simulink model "BaseMotorSimX"  (R2020b)
settings: Solver=VariableStepAuto  StartTime=0.0  StopTime=SimTime  FixedStep=solverTimeStep  RelTol=1e-3
InitFcn:
  | StartupScript
StartFcn:
  | StartupScript
values from neighbouring files (symbols this model uses):
  CF = 372.0    (= 372)    [StartupScript.m]
  Isat = 10.0    (= 10)    [StartupScript.m]
  Kb = 800.0    (= 800)    [StartupScript.m]
  Kdb = 1/(Zerob^2) - Kpb/Poleb    (= 0.414500592554)    [StartupScript.m]
  Kib = 1.0    (= 1)    [StartupScript.m]
  Kmb = 23.4*1e-3    (= 0.0234)    [StartupScript.m]
  Kpb = 2/(Zerob) - 1/Poleb    (= 1.28897849462)    [StartupScript.m]
  PidLim = 1024    [StartupScript.m]
  PidUCGain = 5/1024    (= 0.0048828125)    [StartupScript.m]
  r2d = 180/pi    (= 57.2957795131)    [StartupScript.m]
  sensorGain = 150.0    (= 150)    [StartupScript.m]
  SimStepTime = 1e-3    (= 0.001)    [StartupScript.m]
  Vsat = 18.0    (= 18)    [StartupScript.m]
libraries: cstblocks x3
settings Model: Creator=nisch  LastModifiedBy=nisch

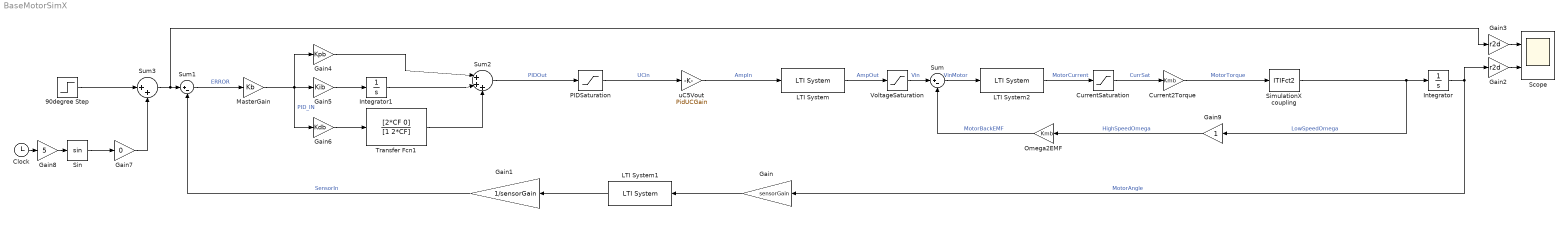
== system BaseMotorSimX ==
  90degree Step : Step  Time=0  After=pi/2  SampleTime=0
  Clock : Clock
  Current2Torque : Gain  Gain=Kmb
  CurrentSaturation : Saturate  UpperLimit=Isat  LowerLimit=-Isat
  Gain : Gain  Gain=sensorGain
  Gain1 : Gain  Gain=1/sensorGain
  Gain2 : Gain  Gain=r2d
  Gain3 : Gain  Gain=r2d
  Gain4 : Gain  Gain=Kpb
  Gain5 : Gain  Gain=Kib
  Gain6 : Gain  Gain=Kdb
  Gain7 : Gain  Gain=0
  Gain8 : Gain  Gain=5
  Gain9 : Gain
  Integrator : Integrator
  Integrator1 : Integrator
  LTI System : cstblocks/LTI System  sys=VoltageAmplifier  IC=[]
  LTI System1 : cstblocks/LTI System  sys=Hs  IC=[]
  LTI System2 : cstblocks/LTI System  sys=Electricalb  IC=[]
  MasterGain : Gain  Gain=Kb
  Omega2EMF : Gain  Gain=Kmb
  PIDSaturation : Saturate  UpperLimit=PidLim  LowerLimit=-PidLim
  Scope : Scope  NumInputPorts=2
  SimulationX coupling : S-Function  FunctionName=ITIFct2  Parameters=ip, port, ts, nIn, nOut  SFunctionDeploymentMode=off  EnableBusSupport=off  mask{ip='localhost', port=4097, ts=SimStepTime, nIn=1, nOut=1}
      mask prompts: ip "Address: ip"; port "Port Number: port [-]"; ts "Communication Step Size: ts [s]"; nIn "Input Vector Dimension (to SimulationX): nIn [-]"; nOut "Output Vector Dimension (from SimulationX): nOut [-]"
      mask help: Coupling Element
  Sin : Trigonometry
  Sum : Sum  Inputs=|+-
  Sum1 : Sum  Inputs=|+-
  Sum2 : Sum  Inputs=|+++
  Sum3 : Sum  Inputs=|++
  Transfer Fcn1 : TransferFcn  Numerator=[2*CF 0]  Denominator=[1 2*CF]
  VoltageSaturation : Saturate  UpperLimit=Vsat  LowerLimit=-Vsat
  uC5Vout : Gain  Gain=PidUCGain
  wires:
  Sum/1 -> LTI System2/1  "VinMotor"
  Omega2EMF/1 -> Sum/2  "MotorBackEMF"
  Sum1/1 -> MasterGain/1  "ERROR"
  Integrator/1 -> Gain2/1, Gain/1  "MotorAngle"
  Gain/1 -> LTI System1/1
  LTI System1/1 -> Gain1/1
  Gain1/1 -> Sum1/2  "SensorIn"
  Gain2/1 -> Scope/2
  Gain3/1 -> Scope/1
  VoltageSaturation/1 -> Sum/1  "Vin"
  MasterGain/1 -> Gain6/1, Gain5/1, Gain4/1  "PID_IN"
  Gain5/1 -> Integrator1/1
  Gain6/1 -> Transfer Fcn1/1
  Sum2/1 -> PIDSaturation/1  "PIDOut"
  Gain4/1 -> Sum2/1
  Integrator1/1 -> Sum2/2
  Transfer Fcn1/1 -> Sum2/3
  LTI System2/1 -> CurrentSaturation/1  "MotorCurrent"
  CurrentSaturation/1 -> Current2Torque/1  "CurrSat"
  Current2Torque/1 -> SimulationX coupling/1  "MotorTorque"
  SimulationX coupling/1 -> Gain9/1, Integrator/1  "LowSpeedOmega"
  Sum3/1 -> Gain3/1, Sum1/1
  90degree Step/1 -> Sum3/1
  Sin/1 -> Gain7/1
  Gain7/1 -> Sum3/2
  Clock/1 -> Gain8/1
  Gain8/1 -> Sin/1
  LTI System/1 -> VoltageSaturation/1  "AmpOut"
  PIDSaturation/1 -> uC5Vout/1  "UCin"
  uC5Vout/1 -> LTI System/1  "AmpIn"
  Gain9/1 -> Omega2EMF/1  "HighSpeedOmega"
